simulink model "AUV_SLIDDING1"  (Simulink 7.6)
settings: Solver=ode5  StartTime=0.0  StopTime=200  FixedStep=.1  RelTol=1e-3
libraries: simulink x4
settings Model: Creator=Comp  LastModifiedBy=HP

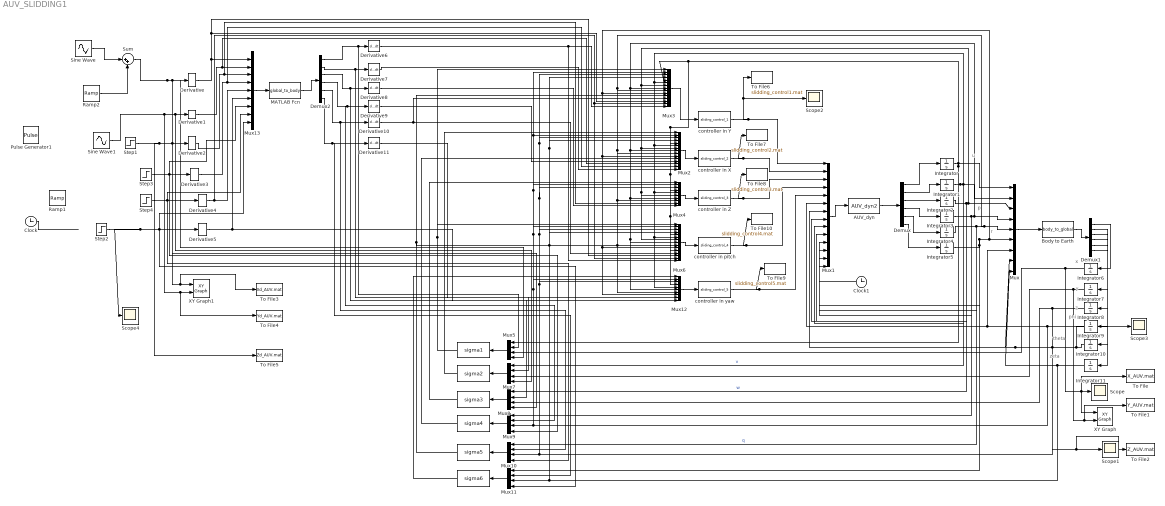
== system AUV_SLIDDING1 ==
  note: u
  note: p
  note: r
  note: x
  note: y
  note: z
  note: phi
  note: theta
  note: zeta
  " " : MATLABFcn  MATLABFcn=sigma6
  "   " : MATLABFcn  MATLABFcn=sigma5
  "    " : MATLABFcn  MATLABFcn=sigma4
  "      " : MATLABFcn  MATLABFcn=sigma3
  "            " : MATLABFcn  MATLABFcn=sigma2
  "                            " : MATLABFcn  MATLABFcn=sigma1
  AUV_dyn : MATLABFcn  MATLABFcn=AUV_dyn2
  Body to Earth : MATLABFcn  MATLABFcn=body_to_global
  Clock : Clock
      settings: Decimation=10
  Clock1 : Clock
      settings: Decimation=10
  Demux : Demux  Outputs=6
  Demux1 : Demux  Outputs=6
  Demux2 : Demux  Outputs=6
  Derivative{,1..11} (12 alike) : Derivative
  Integrator{,1..6,8..11} (11 alike) : Integrator
  Integrator7 : Integrator  InitialCondition=5
  MATLAB Fcn : MATLABFcn  MATLABFcn=global_to_body
  Mux : Mux  Inputs=9
  Mux1 : Mux  Inputs=14
  Mux{5,7..11} (6 alike) : Mux
  Mux12 : Mux  Inputs=10
  Mux13 : Mux  Inputs=9
  Mux2 : Mux  Inputs=15
  Mux3 : Mux  Inputs=15
  Mux4 : Mux  Inputs=10
  Mux6 : Mux  Inputs=15
  Pulse Generator1 : DiscretePulseGenerator  PulseType=Time based  Amplitude=5  Period=20  PulseWidth=50  PhaseDelay=10
  Ramp1 : simulink/Sources/Ramp  SystemSampleTime=-1  slope=0  start=0  X0=0
  Ramp2 : simulink/Sources/Ramp  SystemSampleTime=-1  slope=.25  start=0  X0=0
  Scope{,1..4} (5 alike) : Scope
      Scope2 settings: YMin=-500  YMax=500  SaveName=ScopeData2
      Scope3 settings: SaveName=ScopeData3
      Scope4 settings: SaveName=ScopeData4
  Sine Wave : Sin  Amplitude=2.5  Frequency=.1  SampleTime=0
  Sine Wave1 : Sin  Amplitude=12.5  Frequency=.05  Phase=pi/2  SampleTime=0
  Step1 : Step  Time=0  After=5  SampleTime=0
  Step2 : Step  Time=0  After=0  SampleTime=0
  Step3 : Step  Time=0  After=0  SampleTime=0
  Step4 : Step  Time=0  After=0  SampleTime=0
  Sum : Sum  Inputs=|++
  To File : ToFile  Filename=X_AUV.mat  MatrixName=X  SaveFormat=Timeseries
  To File1 : ToFile  Filename=Y_AUV.mat  MatrixName=Y  SaveFormat=Timeseries
  To File10 : ToFile  Filename=slidding_control4.mat  MatrixName=U4  SaveFormat=Timeseries
  To File2 : ToFile  Filename=Z_AUV.mat  MatrixName=Z  SaveFormat=Timeseries
  To File3 : ToFile  Filename=Xd_AUV.mat  MatrixName=Xd  SaveFormat=Timeseries
  To File4 : ToFile  Filename=Yd_AUV.mat  MatrixName=Yd  SaveFormat=Timeseries
  To File5 : ToFile  Filename=Zd_AUV.mat  MatrixName=Zd  SaveFormat=Timeseries
  To File6 : ToFile  Filename=slidding_control1.mat  MatrixName=U1  SaveFormat=Timeseries
  To File7 : ToFile  Filename=slidding_control2.mat  MatrixName=U2  SaveFormat=Timeseries
  To File8 : ToFile  Filename=slidding_control3.mat  MatrixName=U3  SaveFormat=Timeseries
  To File9 : ToFile  Filename=slidding_control5.mat  MatrixName=U5  SaveFormat=Timeseries
  XY Graph : simulink/Sinks/XY Graph  SystemSampleTime=-1  xmin=0  xmax=60  ymin=-20  ymax=20  st=-1
  XY Graph1 : simulink/Sinks/XY Graph  SystemSampleTime=-1  xmin=-20  xmax=20  ymin=-20  ymax=20  st=-1
  controller in X : MATLABFcn  MATLABFcn=sliding_control_2
  controller in Y : MATLABFcn  MATLABFcn=sliding_control_1
  controller in Z : MATLABFcn  MATLABFcn=sliding_control_3
  controller in pitch : MATLABFcn  MATLABFcn=sliding_control_4
  controller in yaw : MATLABFcn  MATLABFcn=sliding_control_5
  wires:
  AUV_dyn/1 -> Demux/1
  Demux/1 -> Integrator/1
  Demux/2 -> Integrator1/1
  Demux/3 -> Integrator2/1
  Demux/4 -> Integrator3/1
  Demux/5 -> Integrator4/1
  Demux/6 -> Integrator5/1
  Integrator2/1 -> Mux1/10, Mux8/1, Mux/3, Mux3/7, Mux2/7, Mux4/6, Mux6/7  "w"
  Integrator4/1 -> Mux1/12, Mux10/1, Mux/5, Mux3/9, Mux2/9, Mux4/8, Mux6/9, Mux12/7  "q"
  Integrator3/1 -> Mux1/11, Mux9/1, Mux/4, Mux3/8, Mux2/8, Mux4/7, Mux6/8, Mux12/6
  Mux/1 -> Body to Earth/1
  Integrator/1 -> Mux/1, Mux1/8, Mux5/1, Mux3/5, Mux2/5, Mux4/4, Mux6/5, Mux12/4
  Integrator1/1 -> Mux/2, Mux1/9, Mux7/1, Mux3/6, Mux2/6, Mux4/5, Mux6/6, Mux12/5  "v"
  Integrator5/1 -> Mux1/13, Mux11/1, Mux/6, Mux3/10, Mux2/10, Mux6/10, Mux12/8
  Body to Earth/1 -> Demux1/1
  Demux1/1 -> Integrator6/1
  Demux1/2 -> Integrator7/1
  Demux1/3 -> Integrator8/1
  Demux1/4 -> Integrator9/1
  Demux1/5 -> Integrator10/1
  Demux1/6 -> Integrator11/1
  Integrator9/1 -> Mux/7, Mux1/6, Mux3/2, Mux2/2, Mux4/2, Mux6/2, Mux12/2, Mux9/3
  Integrator10/1 -> Mux/8, Mux1/7, Mux10/3, Mux3/3, Mux2/3, Mux4/3, Mux6/3, Mux12/3, Scope3/1
  Integrator11/1 -> Mux/9, Mux11/3, Mux3/4, Mux2/4, Mux6/4
  Mux1/1 -> AUV_dyn/1
  controller in Y/1 -> Mux1/1, To File6/1, Scope2/1
  controller in X/1 -> Mux1/2, To File7/1
  controller in Z/1 -> Mux1/3, To File8/1
  controller in pitch/1 -> Mux1/4, To File10/1
  controller in yaw/1 -> Mux1/5, To File9/1
  Mux5/1 -> "                            "/1
  Integrator6/1 -> Mux5/3, Scope/1, XY Graph/1, To File/1
  Mux7/1 -> "            "/1
  Integrator7/1 -> Mux7/3, XY Graph/2, To File1/1
  Mux8/1 -> "      "/1
  Integrator8/1 -> Mux8/3, Scope1/1, To File2/1
  Mux9/1 -> "    "/1
  Mux10/1 -> "   "/1
  Mux11/1 -> " "/1
  Mux3/1 -> controller in Y/1
  "                            "/1 -> Mux3/1, Mux6/1
  Mux2/1 -> controller in X/1
  Mux4/1 -> controller in Z/1
  Mux6/1 -> controller in pitch/1
  Mux12/1 -> controller in yaw/1
  "   "/1 -> Mux3/11, Mux6/11
  "            "/1 -> Mux2/1
  "    "/1 -> Mux2/11
  "      "/1 -> Mux4/1
  " "/1 -> Mux12/1
  Sum/1 -> Derivative/1, Mux5/4, XY Graph1/1, To File3/1
  Step1/1 -> Derivative2/1, Mux8/4, To File5/1
  Step3/1 -> Derivative3/1, Mux13/7, Mux9/4
  Step4/1 -> Derivative4/1, Mux13/8, Mux10/4
  Step2/1 -> Derivative5/1, Mux13/9, Mux11/4, Scope4/1
  Derivative/1 -> Mux13/1, Mux3/13, Mux6/13
  Derivative1/1 -> Mux13/2, Mux2/13
  Derivative2/1 -> Mux13/3, Mux4/9
  Derivative3/1 -> Mux13/4, Mux2/14
  Derivative4/1 -> Mux13/5, Mux3/14, Mux6/14
  Derivative5/1 -> Mux13/6, Mux12/10
  Mux13/1 -> MATLAB Fcn/1
  Demux2/1 -> Derivative6/1, Mux5/2
  Demux2/2 -> Derivative7/1, Mux7/2
  Demux2/3 -> Derivative8/1, Mux8/2
  Demux2/4 -> Derivative9/1, Mux9/2
  Demux2/5 -> Derivative10/1, Mux10/2
  Demux2/6 -> Derivative11/1, Mux11/2
  Derivative10/1 -> Mux3/12, Mux6/12
  Derivative6/1 -> Mux3/15, Mux6/15
  Derivative9/1 -> Mux2/12
  Derivative7/1 -> Mux2/15
  Derivative8/1 -> Mux4/10
  Derivative11/1 -> Mux12/9
  MATLAB Fcn/1 -> Demux2/1
  Clock/1 -> ?
  Sine Wave1/1 -> Derivative1/1, Mux7/4, XY Graph1/2, To File4/1
  Clock1/1 -> Mux1/14
  Sine Wave/1 -> Sum/1
  Ramp2/1 -> Sum/2
